simulink model "Operating_system_project"  (R2023b)
settings: Solver=VariableStepAuto  StartTime=0.0  StopTime=1.0  RelTol=1e-3
settings Model: Creator=erayd  LastModifiedBy=erayd

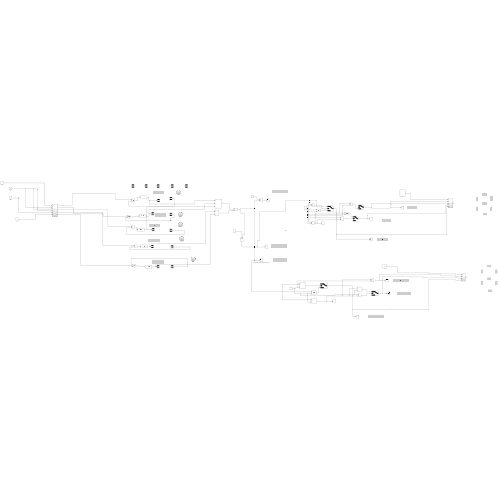
[thumbnail: Simulink's stored preview of the top-level diagram]
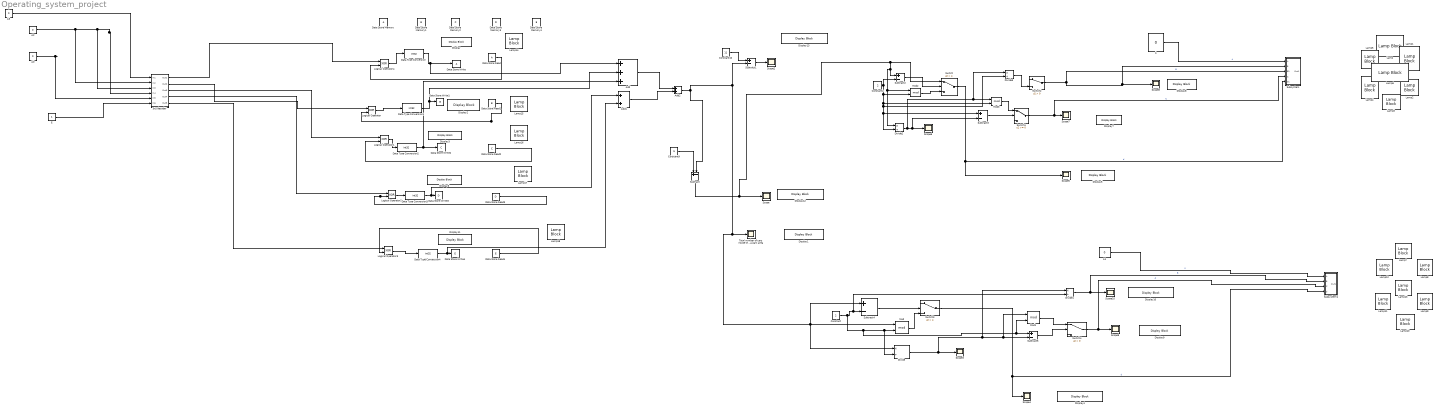
== system Operating_system_project ==
  3x5 decoder : Subsystem
  A{,0..3} (5 alike) : Constant  Value=0
  Add : Sum  Inputs=+++
  Add1 : Sum
  Add2 : Sum
  Constant : Constant  Value=2  OutDataTypeStr=int32
  Constant10 : Constant  Value=11  OutDataTypeStr=int32
  Constant4 : Constant  Value=2  OutDataTypeStr=int32
  Constant9 : Constant  Value=5  OutDataTypeStr=int32
  Data Store Memory : DataStoreMemory  WriteAfterWriteMsg=warning  InitialValue=1  ShowAdditionalParam=off  OutDataTypeStr=int32
  Data Store Memory1 : DataStoreMemory  DataStoreName=B  WriteAfterWriteMsg=warning  ShowAdditionalParam=off  OutDataTypeStr=int32
  Data Store Memory2 : DataStoreMemory  DataStoreName=C  WriteAfterWriteMsg=warning  ShowAdditionalParam=off  OutDataTypeStr=int32
  Data Store Memory3 : DataStoreMemory  DataStoreName=D  WriteAfterWriteMsg=warning  ShowAdditionalParam=off  OutDataTypeStr=int32
  Data Store Memory4 : DataStoreMemory  DataStoreName=E  WriteAfterWriteMsg=warning  ShowAdditionalParam=off  OutDataTypeStr=int32
  Data Store Read : DataStoreRead  IndexOptions=Index vector (dialog)  Indices=1  OutputSizes=1
  Data Store Read1 : DataStoreRead  DataStoreName=B  IndexOptions=Index vector (dialog)  Indices=1  OutputSizes=1
  Data Store Read2 : DataStoreRead  DataStoreName=C  IndexOptions=Index vector (dialog)  Indices=1  OutputSizes=1
  Data Store Read3 : DataStoreRead  DataStoreName=D  IndexOptions=Index vector (dialog)  Indices=1  OutputSizes=1
  Data Store Read4 : DataStoreRead  DataStoreName=E  IndexOptions=Index vector (dialog)  Indices=1  OutputSizes=1
  Data Store Write : DataStoreWrite  IndexOptions=Index vector (dialog)  Indices=1  OutputSizes=1
  Data Store Write1 : DataStoreWrite  DataStoreName=B  IndexOptions=Index vector (dialog)  Indices=1  OutputSizes=1
  Data Store Write2 : DataStoreWrite  DataStoreName=C  IndexOptions=Index vector (dialog)  Indices=1  OutputSizes=1
  Data Store Write3 : DataStoreWrite  DataStoreName=D  IndexOptions=Index vector (dialog)  Indices=1  OutputSizes=1
  Data Store Write4 : DataStoreWrite  DataStoreName=E  IndexOptions=Index vector (dialog)  Indices=1  OutputSizes=1
  Data Type Conversion{,1..4} (5 alike) : DataTypeConversion  OutDataTypeStr=int32  SaturateOnIntegerOverflow=off  RndMeth=Floor
  Display{,1..13} (14 alike) : DisplayBlock  LabelPosition=Hide  Transparency=1
  Divide{,1..3} (4 alike) : Product  Inputs=*/
  E : Constant
  Lamp{,1..13} (14 alike) : LampBlock  LabelPosition=Hide  Icon=Rectangle
  Lamp{14..18} (5 alike) : LampBlock  LabelPosition=Hide
  Logical Operator{,1..4} (5 alike) : Logic  Operator=XOR  AllPortsSameDT=off  OutDataTypeStr=boolean
  Mod{,1..3} (4 alike) : Math  Operator=mod
  Scope{,2..10} (10 alike) : Scope
  Subsystem : Subsystem
  Subsystem1 : Subsystem
  Subtract{,1..5} (6 alike) : Sum  Inputs=+-
  Switch : Switch  Criteria=u2 > Threshold  Threshold=4  SaturateOnIntegerOverflow=off  InputSameDT=off
  Switch1 : Switch  SaturateOnIntegerOverflow=off  InputSameDT=off
  Switch2 : Switch  Criteria=u2 > Threshold  SaturateOnIntegerOverflow=off  InputSameDT=off
  Switch3 : Switch  Criteria=u2 > Threshold  Threshold=4  SaturateOnIntegerOverflow=off  InputSameDT=off
  Switch4 : Switch  Criteria=u2 > Threshold  SaturateOnIntegerOverflow=off  InputSameDT=off
  Total number of cars inside tha park area : Scope
  wires:
  Constant4/1 -> Subtract2/2, Mod2/2, Mod3/2, Divide3/2, Subtract3/1, Divide2/2
  Subtract2/1 -> Switch/2
  Subtract3/1 -> Switch1/2
  Switch/1 -> Subsystem/5(d1), Scope5/1  "d"
  Divide3/1 -> Switch2/3
  Mod2/1 -> Switch/3
  Mod3/1 -> Switch1/1
  Divide2/1 -> Divide3/1, Mod3/1, Subtract3/2, Scope6/1
  Constant/1 -> Mod1/2, Subtract5/1, Divide/2, Mod/2, Divide1/2, Subtract4/2
  Subtract4/1 -> Switch3/2
  Mod/1 -> Switch3/3
  Divide/1 -> Divide1/1, Mod1/1, Subtract5/2, Scope3/1
  Subtract5/1 -> Switch4/2
  Mod1/1 -> Switch4/1
  Switch2/1 -> Subsystem/3(B1), Subsystem/2(B), Scope8/1  "B"
  ? -> ?
  Switch1/1 -> Subsystem/4(C), Scope7/1  "C"
  Switch3/1 -> Scope4/1, Subsystem1/4(d)  "d"
  Divide1/1 -> Subsystem1/2(B), Scope10/1  "B"
  Switch4/1 -> Subsystem1/3(C), Scope9/1  "C"
  Subtract/1 -> Switch/1, Subtract2/1, Mod2/1, Divide2/1, Scope/1
  Add2/1 -> Subtract1/2, Divide/1, Subtract4/1, Mod/1, Total number of cars inside tha park area/1, Subtract/2
  Data Type Conversion/1 -> Add/1, Data Store Write/1
  Data Type Conversion1/1 -> Add/2, Data Store Write1/1
  Logical Operator2/1 -> Data Type Conversion3/1
  Logical Operator4/1 -> Data Type Conversion/1
  Data Store Read4/1 -> Logical Operator3/2
  Data Store Read1/1 -> Logical Operator/2
  Data Type Conversion2/1 -> Add/3, Data Store Write2/1
  Data Store Read3/1 -> Logical Operator2/2
  Constant10/1 -> Subtract1/1
  Add/1 -> Add2/1
  Logical Operator3/1 -> Data Type Conversion4/1
  Data Store Read2/1 -> Logical Operator1/2
  Data Type Conversion3/1 -> Add1/1, Data Store Write3/1
  Subtract1/1 -> Scope2/1
  Data Type Conversion4/1 -> Add1/2, Data Store Write4/1
  Logical Operator1/1 -> Data Type Conversion2/1
  Data Store Read/1 -> Logical Operator4/2
  Logical Operator/1 -> Data Type Conversion1/1
  Constant9/1 -> Subtract/1
  Add1/1 -> Add2/2
  A/1 -> Subsystem/1(A)  "A"
  A1/1 -> Subsystem1/1(A)  "A"
  A0/1 -> 3x5 decoder/5(In5)
  A2/1 -> 3x5 decoder/2(In2), 3x5 decoder/3(In3), 3x5 decoder/4(In4)
  A3/1 -> 3x5 decoder/1(In1)
  E/1 -> 3x5 decoder/6(In6)
  3x5 decoder/1(Out1) -> Logical Operator4/1
  3x5 decoder/2(Out2) -> Logical Operator/1
  3x5 decoder/3(Out3) -> Logical Operator1/1
  3x5 decoder/4(Out4) -> Logical Operator2/1
  3x5 decoder/5(Out5) -> Logical Operator3/1

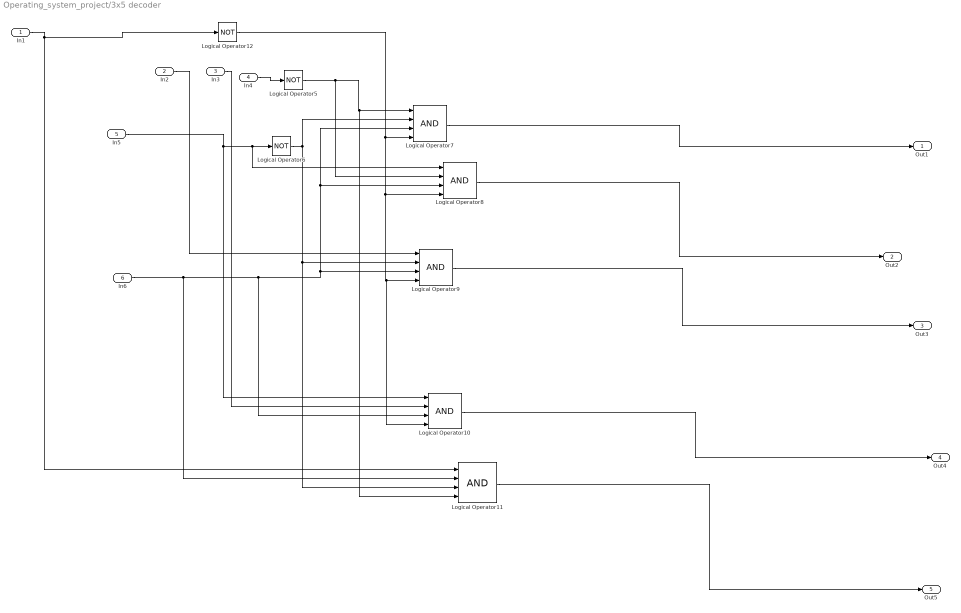
== system Operating_system_project/3x5 decoder ==
  In1 : Inport
  In2 : Inport  Port=2
  In3 : Inport  Port=3
  In4 : Inport  Port=4
  In5 : Inport  Port=5
  In6 : Inport  Port=6
  Logical Operator{7..11} (5 alike) : Logic  Inputs=4  AllPortsSameDT=off  OutDataTypeStr=boolean
  Logical Operator12 : Logic  Operator=NOT  AllPortsSameDT=off  OutDataTypeStr=boolean
  Logical Operator5 : Logic  Operator=NOT  AllPortsSameDT=off  OutDataTypeStr=boolean
  Logical Operator6 : Logic  Operator=NOT  AllPortsSameDT=off  OutDataTypeStr=boolean
  Out1 : Outport
  Out2 : Outport  Port=2
  Out3 : Outport  Port=3
  Out4 : Outport  Port=4
  Out5 : Outport  Port=5
  wires:
  In1/1 -> Logical Operator12/1, Logical Operator11/1
  Logical Operator10/1 -> Out4/1
  Logical Operator7/1 -> Out1/1
  Logical Operator12/1 -> Logical Operator7/4, Logical Operator10/4, Logical Operator9/4, Logical Operator8/4
  In5/1 -> Logical Operator10/1, Logical Operator8/1, Logical Operator6/1
  In6/1 -> Logical Operator11/2, Logical Operator10/3, Logical Operator8/3, Logical Operator7/3, Logical Operator9/3
  In2/1 -> Logical Operator9/1
  Logical Operator9/1 -> Out3/1
  Logical Operator6/1 -> Logical Operator11/3, Logical Operator9/2, Logical Operator7/2
  Logical Operator8/1 -> Out2/1
  Logical Operator5/1 -> Logical Operator8/2, Logical Operator11/4, Logical Operator7/1
  Logical Operator11/1 -> Out5/1
  In3/1 -> Logical Operator10/2
  In4/1 -> Logical Operator5/1

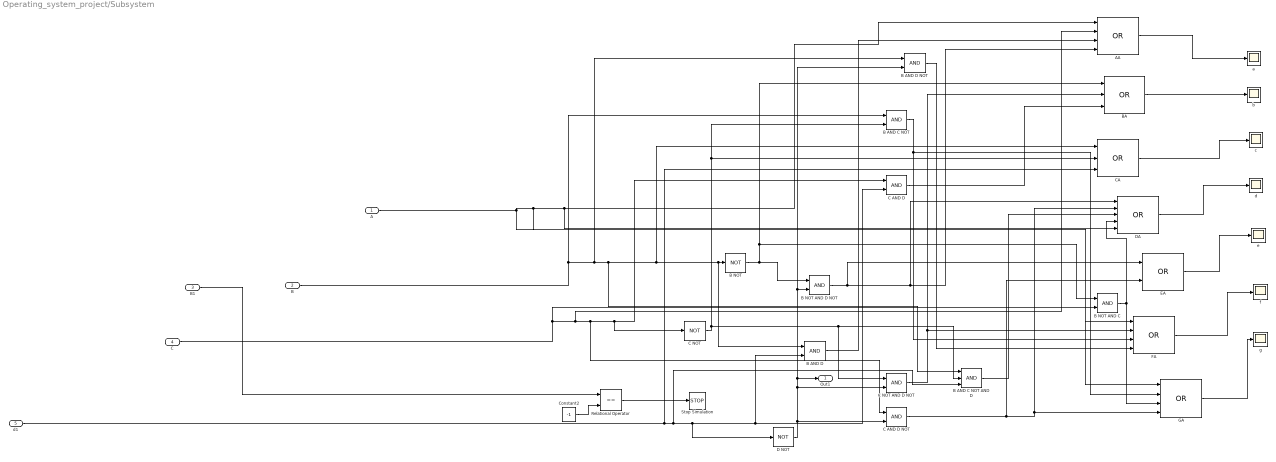
== system Operating_system_project/Subsystem ==
  A : Inport
  B : Inport  Port=2
  B1 : Inport  Port=3
  C : Inport  Port=4
  d1 : Inport  Port=5
  AA : Logic  Operator=OR  Inputs=4  AllPortsSameDT=off  OutDataTypeStr=boolean
  B AND C NOT : Logic  AllPortsSameDT=off  OutDataTypeStr=boolean
  B AND C NOT AND D : Logic  Inputs=3  AllPortsSameDT=off  OutDataTypeStr=boolean
  B AND D : Logic  AllPortsSameDT=off  OutDataTypeStr=boolean
  B AND D NOT : Logic  AllPortsSameDT=off  OutDataTypeStr=boolean
  B NOT : Logic  Operator=NOT  Inputs=4  AllPortsSameDT=off  OutDataTypeStr=boolean
  B NOT AND C : Logic  AllPortsSameDT=off  OutDataTypeStr=boolean
  B NOT AND D NOT : Logic  AllPortsSameDT=off  OutDataTypeStr=boolean
  BA : Logic  Operator=OR  Inputs=3  AllPortsSameDT=off  OutDataTypeStr=boolean
  C AND D : Logic  AllPortsSameDT=off  OutDataTypeStr=boolean
  C AND D NOT : Logic  AllPortsSameDT=off  OutDataTypeStr=boolean
  C NOT : Logic  Operator=NOT  AllPortsSameDT=off  OutDataTypeStr=boolean
  C NOT AND D NOT : Logic  AllPortsSameDT=off  OutDataTypeStr=boolean
  CA : Logic  Operator=OR  Inputs=3  AllPortsSameDT=off  OutDataTypeStr=boolean
  Constant2 : Constant  Value=-1  OutDataTypeStr=int32
  D NOT : Logic  Operator=NOT  Inputs=4  AllPortsSameDT=off  OutDataTypeStr=boolean
  DA : Logic  Operator=OR  Inputs=5  AllPortsSameDT=off  OutDataTypeStr=boolean
  EA : Logic  Operator=OR  AllPortsSameDT=off  OutDataTypeStr=boolean
  FA : Logic  Operator=OR  Inputs=4  AllPortsSameDT=off  OutDataTypeStr=boolean
  GA : Logic  Operator=OR  Inputs=4  AllPortsSameDT=off  OutDataTypeStr=boolean
  Relational Operator : RelationalOperator  Operator===  OutDataTypeStr=boolean  RndMeth=Simplest  InputSameDT=off
  Stop Simulation : Stop
  a : Scope
  b : Scope
  c : Scope
  d : Scope
  e : Scope
  f : Scope
  g : Scope
  Out1 : Outport
  wires:
  B/1 -> B AND C NOT/1, B AND D NOT/1, B AND C NOT AND D/1, CA/1, B AND D/1, B NOT/1
  B AND D/1 -> AA/3
  D NOT/1 -> Out1/1, B AND D NOT/2, B NOT AND D NOT/2, C NOT AND D NOT/2, C AND D NOT/2
  C NOT/1 -> B AND C NOT/2, CA/2, C NOT AND D NOT/1, B AND C NOT AND D/2
  B NOT AND D NOT/1 -> EA/1, DA/1, AA/4
  B NOT/1 -> BA/1, B NOT AND C/1, B NOT AND D NOT/1
  CA/1 -> c/1
  A/1 -> GA/1, DA/5, AA/1, FA/1
  B AND C NOT AND D/1 -> DA/3
  C AND D/1 -> BA/3
  C/1 -> B NOT AND C/2, AA/2, C AND D NOT/1, C NOT/1, C AND D/1
  BA/1 -> b/1
  B AND D NOT/1 -> FA/4
  DA/1 -> d/1
  Relational Operator/1 -> Stop Simulation/1
  AA/1 -> a/1
  C AND D NOT/1 -> EA/2, GA/4, DA/2
  B NOT AND C/1 -> DA/4, GA/3
  C NOT AND D NOT/1 -> FA/2, BA/2
  FA/1 -> f/1
  EA/1 -> e/1
  GA/1 -> g/1
  B AND C NOT/1 -> GA/2, FA/3
  d1/1 -> CA/3, B AND C NOT AND D/3, C AND D/2, B AND D/2, D NOT/1
  Constant2/1 -> Relational Operator/2
  B1/1 -> Relational Operator/1

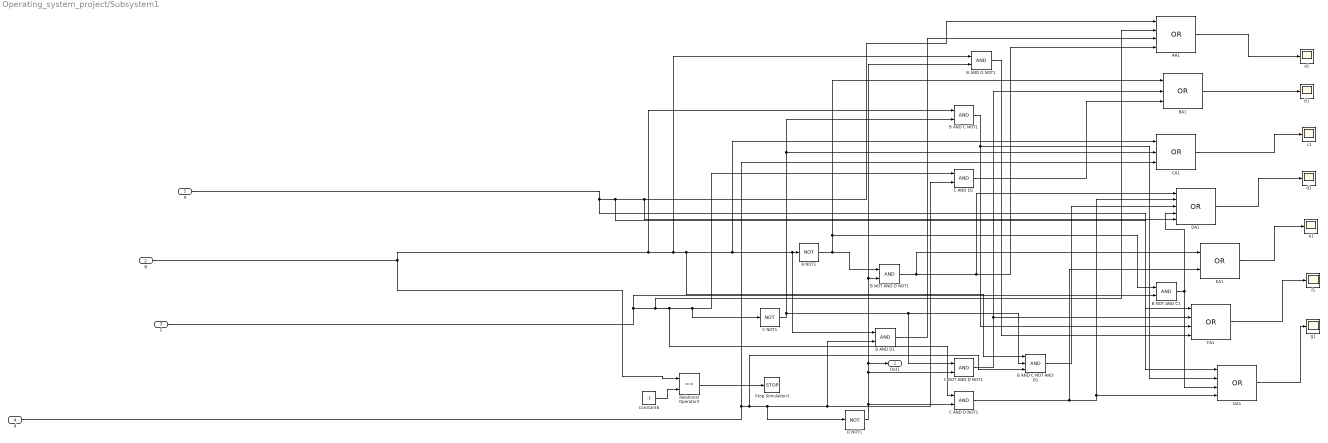
== system Operating_system_project/Subsystem1 ==
  A : Inport
  B : Inport  Port=2
  C : Inport  Port=3
  d : Inport  Port=4
  AA1 : Logic  Operator=OR  Inputs=4  AllPortsSameDT=off  OutDataTypeStr=boolean
  B AND C NOT AND D1 : Logic  Inputs=3  AllPortsSameDT=off  OutDataTypeStr=boolean
  B AND C NOT1 : Logic  AllPortsSameDT=off  OutDataTypeStr=boolean
  B AND D NOT1 : Logic  AllPortsSameDT=off  OutDataTypeStr=boolean
  B AND D1 : Logic  AllPortsSameDT=off  OutDataTypeStr=boolean
  B NOT AND C1 : Logic  AllPortsSameDT=off  OutDataTypeStr=boolean
  B NOT AND D NOT1 : Logic  AllPortsSameDT=off  OutDataTypeStr=boolean
  B NOT1 : Logic  Operator=NOT  Inputs=4  AllPortsSameDT=off  OutDataTypeStr=boolean
  BA1 : Logic  Operator=OR  Inputs=3  AllPortsSameDT=off  OutDataTypeStr=boolean
  C AND D NOT1 : Logic  AllPortsSameDT=off  OutDataTypeStr=boolean
  C AND D1 : Logic  AllPortsSameDT=off  OutDataTypeStr=boolean
  C NOT AND D NOT1 : Logic  AllPortsSameDT=off  OutDataTypeStr=boolean
  C NOT1 : Logic  Operator=NOT  AllPortsSameDT=off  OutDataTypeStr=boolean
  CA1 : Logic  Operator=OR  Inputs=3  AllPortsSameDT=off  OutDataTypeStr=boolean
  Constant6 : Constant  Value=-1  OutDataTypeStr=int32
  D NOT1 : Logic  Operator=NOT  Inputs=4  AllPortsSameDT=off  OutDataTypeStr=boolean
  DA1 : Logic  Operator=OR  Inputs=5  AllPortsSameDT=off  OutDataTypeStr=boolean
  EA1 : Logic  Operator=OR  AllPortsSameDT=off  OutDataTypeStr=boolean
  FA1 : Logic  Operator=OR  Inputs=4  AllPortsSameDT=off  OutDataTypeStr=boolean
  GA1 : Logic  Operator=OR  Inputs=4  AllPortsSameDT=off  OutDataTypeStr=boolean
  Relational Operator3 : RelationalOperator  Operator===  OutDataTypeStr=boolean  RndMeth=Simplest  InputSameDT=off
  Stop Simulation3 : Stop
  a1 : Scope
  b1 : Scope
  c1 : Scope
  d1 : Scope
  e1 : Scope
  f1 : Scope
  g1 : Scope
  Out1 : Outport
  wires:
  BA1/1 -> b1/1
  B NOT AND C1/1 -> DA1/4, GA1/3
  C NOT1/1 -> B AND C NOT1/2, CA1/2, C NOT AND D NOT1/1, B AND C NOT AND D1/2
  B AND C NOT AND D1/1 -> DA1/3
  Constant6/1 -> Relational Operator3/2
  B/1 -> Relational Operator3/1, B AND C NOT1/1, B AND D NOT1/1, B AND C NOT AND D1/1, CA1/1, B AND D1/1, B NOT1/1
  d/1 -> CA1/3, B AND C NOT AND D1/3, C AND D1/2, B AND D1/2, D NOT1/1
  A/1 -> FA1/1, GA1/1, DA1/5, AA1/1
  D NOT1/1 -> Out1/1, B AND D NOT1/2, B NOT AND D NOT1/2, C NOT AND D NOT1/2, C AND D NOT1/2
  B AND C NOT1/1 -> GA1/2, FA1/3
  CA1/1 -> c1/1
  DA1/1 -> d1/1
  B NOT AND D NOT1/1 -> EA1/1, DA1/1, AA1/4
  AA1/1 -> a1/1
  C/1 -> B NOT AND C1/2, AA1/2, C AND D NOT1/1, C NOT1/1, C AND D1/1
  C AND D1/1 -> BA1/3
  B NOT1/1 -> BA1/1, B NOT AND C1/1, B NOT AND D NOT1/1
  B AND D1/1 -> AA1/3
  Relational Operator3/1 -> Stop Simulation3/1
  GA1/1 -> g1/1
  B AND D NOT1/1 -> FA1/4
  C NOT AND D NOT1/1 -> FA1/2, BA1/2
  FA1/1 -> f1/1
  C AND D NOT1/1 -> EA1/2, GA1/4, DA1/2
  EA1/1 -> e1/1
